simulink model "rollobserver"  (R2016a)
settings: Solver=VariableStepAuto  StartTime=0.0  StopTime=20  RelTol=1e-3
libraries: simulink x1
settings Model: Creator=GusBus  LastModifiedBy=GusBus

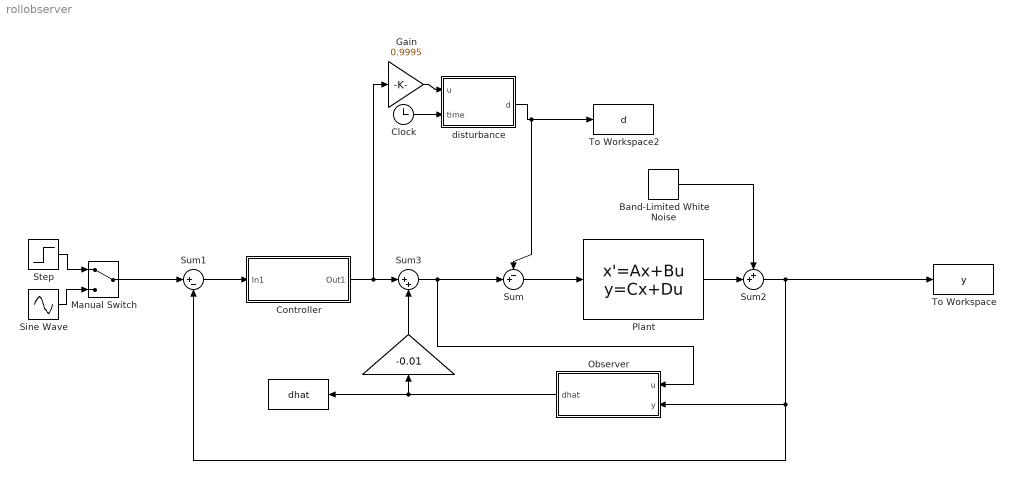
== system rollobserver ==
  " " : Gain  Gain=-0.01
  "  " : ToWorkspace  VariableName=dhat  SampleTime=-1
  Band-Limited White Noise : simulink/Sources/Band-Limited White Noise  Cov=[0.1]*0.0001  Ts=0.1  seed=[23341]
  Clock : Clock
  Controller : Subsystem
  Gain : Gain  Gain=0.9995
  Manual Switch : ManualSwitch
  Observer : Subsystem
  Plant : StateSpace  A=0  B=1/0.02508  D=0  X0=0
  Sine Wave : Sin  SampleTime=0
  Step : Step  SampleTime=0
  Sum : Sum  Inputs=-+|
  Sum1 : Sum  Inputs=|+-
  Sum2 : Sum  Inputs=++|
  Sum3 : Sum  Inputs=|++
  To Workspace : ToWorkspace  VariableName=y  SampleTime=-1
  To Workspace2 : ToWorkspace  VariableName=d  SampleTime=-1
  disturbance : MATLAB Function  TreatAsAtomicUnit=on
  wires:
  Controller/1(Out1) -> Gain/1, Sum3/1
  Sum1/1 -> Controller/1(In1)
  Manual Switch/1 -> Sum1/1
  Sine Wave/1 -> Manual Switch/2
  Step/1 -> Manual Switch/1
  Gain/1 -> disturbance/1(u)
  Plant/1 -> Sum2/2
  Sum2/1 -> Sum1/2, Observer/2("y "), To Workspace/1
  Clock/1 -> disturbance/2(time)
  Sum/1 -> Plant/1
  Sum3/1 -> Observer/1("u "), Sum/2
  Observer/1(dhat) -> " "/1, "  "/1
  disturbance/1(d) -> To Workspace2/1, Sum/1
  Band-Limited White Noise/1 -> Sum2/1
  " "/1 -> Sum3/2

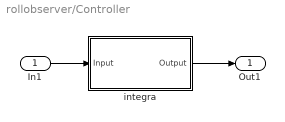
== system rollobserver/Controller ==
  In1 : Inport
  integra : Subsystem
  Out1 : Outport
  wires:
  integra/1(Output) -> Out1/1
  In1/1 -> integra/1(Input)

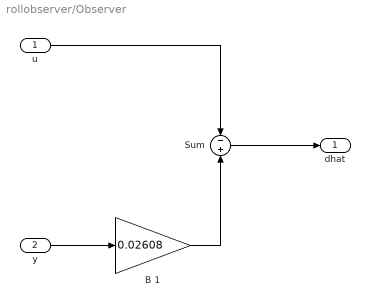
== system rollobserver/Observer ==
  "u " : Inport
  "y " : Inport  Port=2
  B 1 : Gain  Gain=0.02608
  Sum : Sum  Inputs=-|+
  dhat : Outport
  wires:
  "u "/1 -> Sum/1
  "y "/1 -> B 1/1
  B 1/1 -> Sum/2
  Sum/1 -> dhat/1

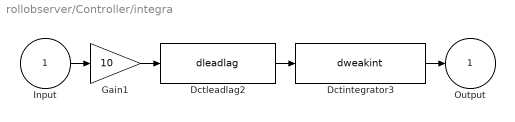
== system rollobserver/Controller/integra ==
  Input : Inport
  Dctintegrator3 : S-Function  FunctionName=dweakint  Parameters=f_num, 0.001  SFunctionDeploymentMode=off  EnableBusSupport=off  mask(dctools){f_num=1}
      mask prompts: f_num "Zero [Hz]"
      mask help: This block implements a discrete time weak integrator filter.
      mask Display: disp('DCT integrator')
  Dctleadlag2 : S-Function  FunctionName=dleadlag  Parameters=f_num, f_den, 0.001  SFunctionDeploymentMode=off  EnableBusSupport=off  mask(dctools){f_num=100, f_den=3.3333}
      mask prompts: f_num "Zero [Hz]"; f_den "Pole [Hz]"
      mask help: This block implements a discrete time leadlag filter.
      mask Display: disp('DCT leadlag')
  Gain1 : Gain  Gain=10  SaturateOnIntegerOverflow=on  OutDataTypeStr=Inherit: Same as input  ParamDataTypeStr=Inherit: Same as input
  Output : Outport
  wires:
  Input/1 -> Gain1/1
  Gain1/1 -> Dctleadlag2/1
  Dctleadlag2/1 -> Dctintegrator3/1
  Dctintegrator3/1 -> Output/1

== matlab function rollobserver/disturbance ==
  data: u input; d output; time input
function d  = disturbance(u,time)
%#codegen
d=0;
if time >= 5.5
    d = u;
end
